simulink model "forceFeilds_sim"  (R2024b)
settings: Solver=FixedStepDiscrete  StartTime=0.0  StopTime=inf  FixedStep=0.001  RelTol=1e-3
libraries: PhanTorque_3Dof_Library_64Bits x2, simulink x1
settings Model: Creator=carlos.aldana  LastModifiedBy=Wassim
settings SolverCC: AlgebraicLoopSolver=TrustRegion
settings DataIOCC: LimitDataPoints=on  SaveFormat=Array  ReturnWorkspaceOutputs=off
settings OptimizationCC: BlockReduction=off  BooleanDataType=off  LifeSpan=inf
settings DebuggingCC: SaveWithParameterizedLinksMsg=none  UnderspecifiedInitializationDetection=Classic  MergeDetectMultiDrivingBlocksExec=none  SignalResolutionControl=TryResolveAllWithWarning  UnconnectedInputMsg=warning  UnconnectedOutputMsg=warning  UnconnectedLineMsg=warning  AllowSymbolicDim=off  SFUnexpectedBacktrackingDiag=warning  SFNoUnconditionalDefaultTransitionDiag=warning  SFExecutionAtInitializationDiag=none  ArithmeticOperatorsInVariantConditions=warning
settings HardwareCC: ProdBitPerPointer=32  ProdBitPerSizeT=32  ProdBitPerPtrDiffT=32  ProdLargestAtomicFloat=None  ProdIntDivRoundTo=Undefined  ProdEndianess=Unspecified  ProdWordSize=32  ProdHWDeviceType=32-bit Generic  TargetUnknown=on
settings ModelReferenceCC: EnableRefExpFcnMdlSchedulingChecks=on  PropagateSignalLabelsOutOfModel=off
settings SFSimCC: SimUseLocalCustomCode=off  CustomCodeUndefinedFunction=UseInterfaceOnly
settings RTWCC: RTWUseLocalCustomCode=off  GPUComputeCapability=3.5  DLArmComputeVersion=19.05
settings CodeAppCC: StateflowObjectComments=on
settings GRTTargetCC: TargetLangStandard=C89/C90 (ANSI)
settings ConfigComp: CovMetricSettings=dw  CovSaveCumulativeToWorkspaceVar=on  CovSaveSingleToWorkspaceVar=on  CovExternalEMLEnable=off  CovSFcnEnable=off

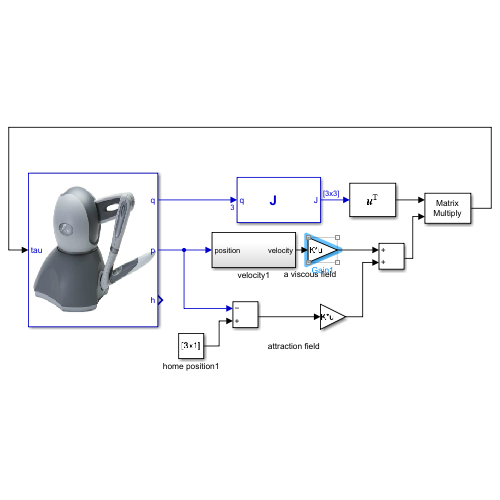
[thumbnail: Simulink's stored preview of the top-level diagram]
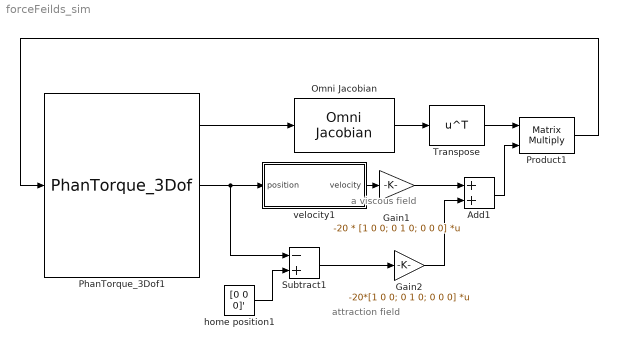
== system forceFeilds_sim ==
  note: attraction field
  note: a viscous field
  Add1 : Sum
  Gain1 : Gain  Gain=-20 * [1 0 0; 0 1 0; 0 0 0]  Multiplication=Matrix(K*u)
  Gain2 : Gain  Gain=-20*[1 0 0; 0 1 0; 0 0 0]  Multiplication=Matrix(K*u)
  Omni Jacobian : PhanTorque_3Dof_Library_64Bits/Omni Jacobian  SystemSampleTime=-1  VariantActivationTime=update diagram  AllowFlexibleInterface=on  Latency=0  AutoFrameSizeCalculation=off
  PhanTorque_3Dof1 : PhanTorque_3Dof_Library_64Bits/PhanTorque_3Dof  Haptic_Name='Default Device'
  Product1 : Product  Multiplication=Matrix(*)
  Subtract1 : Sum  Inputs=-+
  Transpose : Math  Operator=transpose  SignedPower=on
  home position1 : Constant  Value=[0 0 0]'
  velocity1 : Subsystem
  wires:
  PhanTorque_3Dof1/1 -> Omni Jacobian/1
  Product1/1 -> PhanTorque_3Dof1/1
  Add1/1 -> Product1/2
  PhanTorque_3Dof1/2 -> Subtract1/1, velocity1/1(position)
  velocity1/1(velocity) -> Gain1/1
  Gain1/1 -> Add1/1
  Gain2/1 -> Add1/2
  Subtract1/1 -> Gain2/1
  home position1/1 -> Subtract1/2
  Omni Jacobian/1 -> Transpose/1
  Transpose/1 -> Product1/1

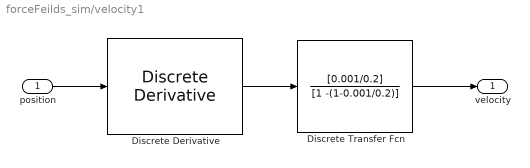
== system forceFeilds_sim/velocity1 ==
  position : Inport
  Discrete Derivative : simulink/Discrete/Discrete Derivative  gainval=1.0  ICPrevScaledInput=0.0  OutMin=[]  OutMax=[]  OutDataType=fixdt(1, 16)  OutScaling=2^-10  DoSatur=off
  Discrete Transfer Fcn : DiscreteTransferFcn  Numerator=[0.001/0.2]  Denominator=[1 -(1-0.001/0.2)]
  velocity : Outport  VectorParamsAs1DForOutWhenUnconnected=off
  wires:
  position/1 -> Discrete Derivative/1
  Discrete Derivative/1 -> Discrete Transfer Fcn/1
  Discrete Transfer Fcn/1 -> velocity/1
